simulink subsystem "Line"  (R2020b)
settings: Solver=VariableStepAuto  StartTime=0.0  StopTime=10.0  RelTol=1e-3
undefined symbols (not defined in the file): DCHigh, DCLow
libraries: fl_lib x2
settings Model: Creator=cao2851  LastModifiedBy=cao2851

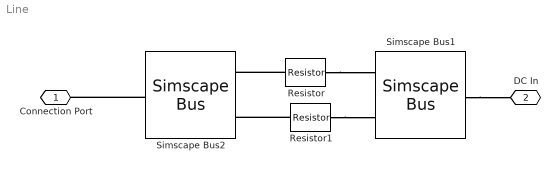
== system Line ==
  Resistor : fl_lib/Electrical/Electrical Elements/Resistor  R=1 Ohm  i_specify=off  i_priority=None  i=0 A  i_nominal_specify=off  i_nominal_unit=A  i_nominal_value=1  v_specify=off  v_priority=None  v=0 V  v_nominal_specify=off  v_nominal_unit=V  v_nominal_value=1
  Resistor1 : fl_lib/Electrical/Electrical Elements/Resistor  R=1 Ohm  i_specify=off  i_priority=None  i=0 A  i_nominal_specify=off  i_nominal_unit=A  i_nominal_value=1  v_specify=off  v_priority=None  v=0 V  v_nominal_specify=off  v_nominal_unit=V  v_nominal_value=1
  Simscape Bus1 : SimscapeBus  HierarchyStrings=DCHigh;DCLow
  Simscape Bus2 : SimscapeBus  HierarchyStrings=DCHigh;DCLow
  Connection Port : PMIOPort  Side=Left
  DC In : PMIOPort  Port=2  Side=Right
  connections:
  Simscape Bus2/RConn1 -- Connection Port/RConn1
  Simscape Bus1/RConn1 -- DC In/RConn1
  Resistor/LConn1 -- Simscape Bus2/LConn1
  Resistor/RConn1 -- Simscape Bus1/LConn1
  Resistor1/LConn1 -- Simscape Bus2/LConn2
  Resistor1/RConn1 -- Simscape Bus1/LConn2
